simulink model "uav_dan"  (R2016b)
settings: Solver=ode4  StartTime=0.0  StopTime=40  FixedStep=0.001  RelTol=1e-3
libraries: simulink x3
settings Model: Creator=Administrator  LastModifiedBy=Administrator

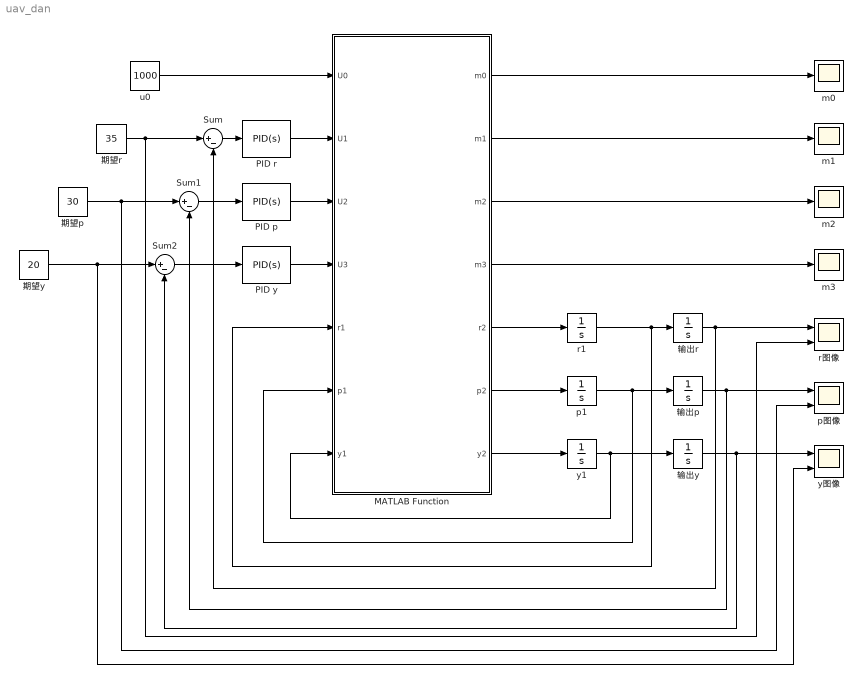
== system uav_dan ==
  MATLAB Function : MATLAB Function  TreatAsAtomicUnit=on
  PID p : simulink/Continuous/PID Controller  Controller=PID  TimeDomain=Continuous-time  SampleTime=-1  IntegratorMethod=Forward Euler  FilterMethod=Forward Euler  Form=Parallel  UseFilter=on  ControllerParametersSource=internal  P=15  I=3  D=5  N=100  InitialConditionSource=internal  InitialConditionForIntegrator=0  InitialConditionForFilter=0  ExternalReset=none  LimitOutput=on  UpperSaturationLimit=200  LowerSaturationLimit=-200  LinearizeAsGain=on  AntiWindupMode=none  Kb=1  TrackingMode=off  Kt=1  PParamMin=[]  PParamMax=[]  IParamMin=[]  IParamMax=[]  DParamMin=[]  DParamMax=[]  NParamMin=[]  NParamMax=[]  KbParamMin=[]  KbParamMax=[]  KtParamMin=[]  KtParamMax=[]  POutMin=[]  POutMax=[]  IOutMin=[]  IOutMax=[]  DOutMin=[]  DOutMax=[]  NOutMin=[]  NOutMax=[]  KbOutMin=[]  KbOutMax=[]  KtOutMin=[]  KtOutMax=[]  IntegratorOutMin=[]  IntegratorOutMax=[]  FilterOutMin=[]  FilterOutMax=[]  SumOutMin=[]  SumOutMax=[]  SumI1OutMin=[]  SumI1OutMax=[]  SumI2OutMin=[]  SumI2OutMax=[]  SumI3OutMin=[]  SumI3OutMax=[]  SumDOutMin=[]  SumDOutMax=[]  SaturationOutMin=[]  SaturationOutMax=[]  IntegratorContinuousStateAttributes=''  IntegratorStateMustResolveToSignalObject=off  IntegratorRTWStateStorageClass=Auto  FilterContinuousStateAttributes=''  FilterStateMustResolveToSignalObject=off  FilterRTWStateStorageClass=Auto  DifferentiatorICPrevScaledInput=0  DifferentiatorOutMin=[]  DifferentiatorOutMax=[]
  PID r : simulink/Continuous/PID Controller  Controller=PID  TimeDomain=Continuous-time  SampleTime=-1  IntegratorMethod=Forward Euler  FilterMethod=Forward Euler  Form=Parallel  UseFilter=on  ControllerParametersSource=internal  P=15  I=3  D=5  N=100  InitialConditionSource=internal  InitialConditionForIntegrator=0  InitialConditionForFilter=0  ExternalReset=none  LimitOutput=on  UpperSaturationLimit=100  LowerSaturationLimit=-100  LinearizeAsGain=on  AntiWindupMode=none  Kb=1  TrackingMode=off  Kt=1  PParamMin=[]  PParamMax=[]  IParamMin=[]  IParamMax=[]  DParamMin=[]  DParamMax=[]  NParamMin=[]  NParamMax=[]  KbParamMin=[]  KbParamMax=[]  KtParamMin=[]  KtParamMax=[]  POutMin=[]  POutMax=[]  IOutMin=[]  IOutMax=[]  DOutMin=[]  DOutMax=[]  NOutMin=[]  NOutMax=[]  KbOutMin=[]  KbOutMax=[]  KtOutMin=[]  KtOutMax=[]  IntegratorOutMin=[]  IntegratorOutMax=[]  FilterOutMin=[]  FilterOutMax=[]  SumOutMin=[]  SumOutMax=[]  SumI1OutMin=[]  SumI1OutMax=[]  SumI2OutMin=[]  SumI2OutMax=[]  SumI3OutMin=[]  SumI3OutMax=[]  SumDOutMin=[]  SumDOutMax=[]  SaturationOutMin=[]  SaturationOutMax=[]  IntegratorContinuousStateAttributes=''  IntegratorStateMustResolveToSignalObject=off  IntegratorRTWStateStorageClass=Auto  FilterContinuousStateAttributes=''  FilterStateMustResolveToSignalObject=off  FilterRTWStateStorageClass=Auto  DifferentiatorICPrevScaledInput=0  DifferentiatorOutMin=[]  DifferentiatorOutMax=[]
  PID y : simulink/Continuous/PID Controller  Controller=PID  TimeDomain=Continuous-time  SampleTime=-1  IntegratorMethod=Forward Euler  FilterMethod=Forward Euler  Form=Parallel  UseFilter=on  ControllerParametersSource=internal  P=9  I=2  D=3  N=100  InitialConditionSource=internal  InitialConditionForIntegrator=0  InitialConditionForFilter=0  ExternalReset=none  LimitOutput=on  UpperSaturationLimit=200  LowerSaturationLimit=-200  LinearizeAsGain=on  AntiWindupMode=none  Kb=1  TrackingMode=off  Kt=1  PParamMin=[]  PParamMax=[]  IParamMin=[]  IParamMax=[]  DParamMin=[]  DParamMax=[]  NParamMin=[]  NParamMax=[]  KbParamMin=[]  KbParamMax=[]  KtParamMin=[]  KtParamMax=[]  POutMin=[]  POutMax=[]  IOutMin=[]  IOutMax=[]  DOutMin=[]  DOutMax=[]  NOutMin=[]  NOutMax=[]  KbOutMin=[]  KbOutMax=[]  KtOutMin=[]  KtOutMax=[]  IntegratorOutMin=[]  IntegratorOutMax=[]  FilterOutMin=[]  FilterOutMax=[]  SumOutMin=[]  SumOutMax=[]  SumI1OutMin=[]  SumI1OutMax=[]  SumI2OutMin=[]  SumI2OutMax=[]  SumI3OutMin=[]  SumI3OutMax=[]  SumDOutMin=[]  SumDOutMax=[]  SaturationOutMin=[]  SaturationOutMax=[]  IntegratorContinuousStateAttributes=''  IntegratorStateMustResolveToSignalObject=off  IntegratorRTWStateStorageClass=Auto  FilterContinuousStateAttributes=''  FilterStateMustResolveToSignalObject=off  FilterRTWStateStorageClass=Auto  DifferentiatorICPrevScaledInput=0  DifferentiatorOutMin=[]  DifferentiatorOutMax=[]
  Sum : Sum  Inputs=|+-
  Sum1 : Sum  Inputs=|+-
  Sum2 : Sum  Inputs=|+-
  m{0..3} (4 alike) : Scope
  p1 : Integrator
  p图像 : Scope  NumInputPorts=2
  r1 : Integrator
  r图像 : Scope  NumInputPorts=2
  u0 : Constant  Value=1000
  y1 : Integrator
  y图像 : Scope  NumInputPorts=2
  期望p : Constant  Value=30
  期望r : Constant  Value=35
  期望y : Constant  Value=20
  输出p : Integrator
  输出r : Integrator
  输出y : Integrator
  wires:
  MATLAB Function/5(r2) -> r1/1
  r1/1 -> MATLAB Function/5(r1), 输出r/1
  期望r/1 -> r图像/2, Sum/1
  Sum/1 -> PID r/1
  MATLAB Function/6(p2) -> p1/1
  p1/1 -> MATLAB Function/6(p1), 输出p/1
  MATLAB Function/7(y2) -> y1/1
  y1/1 -> MATLAB Function/7(y1), 输出y/1
  PID r/1 -> MATLAB Function/2(U1)
  期望p/1 -> p图像/2, Sum1/1
  Sum1/1 -> PID p/1
  PID p/1 -> MATLAB Function/3(U2)
  期望y/1 -> y图像/2, Sum2/1
  Sum2/1 -> PID y/1
  PID y/1 -> MATLAB Function/4(U3)
  u0/1 -> MATLAB Function/1(U0)
  MATLAB Function/1(m0) -> m0/1
  MATLAB Function/2(m1) -> m1/1
  MATLAB Function/3(m2) -> m2/1
  MATLAB Function/4(m3) -> m3/1
  输出r/1 -> Sum/2, r图像/1
  输出p/1 -> p图像/1, Sum1/2
  输出y/1 -> y图像/1, Sum2/2

== matlab function uav_dan/MATLAB Function ==
  data: U0 input; m0 output; U1 input; U2 input; m1 output; m2 output; m3 output; r2 output; p2 output; y2 output; U3 input; r1 input; p1 input; y1 input
function [m0, m1, m2, m3, r2, p2, y2] = fcn(U0, U1, U2, U3, r1, p1, y1)
l = 0.23;
Ix = 0.00482;
Iy = 0.00482;
Iz = 0.01865;


r2  = (l*U1 + p1*y1*(Ix - Iz))/Iy;
p2  = (l*U2 + r1*y1*(Iz - Iy))/Ix;
y2  = (U3 + r1*y1*(Iy - Ix))/Iz;


m0 = U0 + U1 - U2 - U3;%%左前
m1 = U0 - U1 - U2 + U3;%%右前
m2 = U0 + U1 + U2 + U3;%%左后
m3 = U0 - U1 + U2 - U3;%%右后

end
